simulink model "ROME_9DOF"  (R2026a)
settings: Solver=FixedStepDiscrete  StopTime=T_scaled  FixedStep=dt_9dof  EnableMultiTasking=on
PostLoadFcn:
  | define_constants
model workspace (MAT data in the model file):
  dddwad = 1
values from neighbouring files (symbols this model uses):
  alphas = [5.49778714378 3.92699081699 2.35619449019 0.785398163397]    [9-24-26-15-33_Case_1_data.mat]    (also in define_constants.m = [deg2rad(315), deg2rad(225), deg2rad(135), deg2rad(45)]; scaled_factor_0.1_scenario1.mat; scaled_factor_1.0_scenario1_semimajor0.5.mat; scaled_factor_1.0_scenario1_semimajor10.mat)
  arm_home = [-0.0523598775598 2.21656815003 -0.174532925199 0 -0.471238898038 0]    [9-24-26-15-33_Case_1_data.mat]    (also in define_constants.m = deg2rad([-3.0; -53.0; -10.0; 0.0; -27.0; 0.0]); scaled_factor_0.1_scenario1.mat = [0 -0.5 0.9 0 0.7 0]; scaled_factor_1.0_scenario1_semimajor0.5.mat = [0 -0.5 0.9 0 0.7 0]; scaled_factor_1.0_scenario1_semimajor10.mat = [0 -0.5 0.9 0 0.7 0])
  dist_scale = 0.5    [9-24-26-15-33_Case_1_data.mat]    (also in define_constants.m; scaled_factor_0.1_scenario1.mat = 0.1; scaled_factor_1.0_scenario1_semimajor0.5.mat = 1; scaled_factor_1.0_scenario1_semimajor10.mat = 1)
  dt_9dof = 0.05    [9-24-26-15-33_Case_1_data.mat]    (also in define_constants.m; scaled_factor_0.1_scenario1.mat; scaled_factor_1.0_scenario1_semimajor0.5.mat; scaled_factor_1.0_scenario1_semimajor10.mat)
  elements = [1.4 0.5 0 0 0 0]    [9-24-26-15-33_Case_1_data.mat]    (also in define_constants.m = [1.4, 0.5, 0, 0, 0, 0]; scaled_factor_0.1_scenario1.mat; scaled_factor_1.0_scenario1_semimajor0.5.mat = [0.5 0.5 0 0 0 0]; scaled_factor_1.0_scenario1_semimajor10.mat = [10 0.5 0 0 0 0])
  EnableHardware = 1    [9-24-26-15-33_Case_1_data.mat]    (also in define_constants.m = 0; scaled_factor_0.1_scenario1.mat; scaled_factor_1.0_scenario1_semimajor0.5.mat = 0; scaled_factor_1.0_scenario1_semimajor10.mat = 0)
  EnableMotive = 0    [9-24-26-15-33_Case_1_data.mat]    (also in define_constants.m; scaled_factor_0.1_scenario1.mat; scaled_factor_1.0_scenario1_semimajor0.5.mat; scaled_factor_1.0_scenario1_semimajor10.mat)
  l = 0.35    [9-24-26-15-33_Case_1_data.mat]    (also in define_constants.m; scaled_factor_0.1_scenario1.mat; scaled_factor_1.0_scenario1_semimajor0.5.mat; scaled_factor_1.0_scenario1_semimajor10.mat)
  max_rpm = 60    [9-24-26-15-33_Case_1_data.mat]    (also in define_constants.m = 120)
  mu = 1    [9-24-26-15-33_Case_1_data.mat]    (also in define_constants.m; scaled_factor_0.1_scenario1.mat; scaled_factor_1.0_scenario1_semimajor0.5.mat; scaled_factor_1.0_scenario1_semimajor10.mat)
  par = [0 0 0 0]    [9-24-26-15-33_Case_1_data.mat]    (also in define_constants.m; scaled_factor_0.1_scenario1.mat; scaled_factor_1.0_scenario1_semimajor0.5.mat; scaled_factor_1.0_scenario1_semimajor10.mat)
  q0_9dof = [0.677771808272 -0.00755462438616 -3.12693488796 -0.0377021119487 2.24411564415 -0.258737272647 -2.32231542275e-11 -0.414582044708 -0.0230443461837]    [9-24-26-15-33_Case_1_data.mat]    (also in define_constants.m = ik9_warm_start(q0_9dof, p_ref0, u_ref0); scaled_factor_0.1_scenario1.mat = [0.419801308893 0.000544930315419 0.0507789134473 -0.0492210; scaled_factor_1.0_scenario1_semimajor0.5.mat = [0.597187365937 -0.000238669500436 0.0496562814685 -0.050343; scaled_factor_1.0_scenario1_semimajor10.mat = [5.22393486573 -0.00540150303984 0.0379419048008 -0.06205809)
  qd0_9dof = [0 0 0 0 0 0 0 0 0]    [9-24-26-15-33_Case_1_data.mat]    (also in define_constants.m = zeros(9,1); scaled_factor_0.1_scenario1.mat = [-0.00873270617541 7.41536811609 7.95269754129 7.95269754129; scaled_factor_1.0_scenario1_semimajor0.5.mat = [0.00054251154028 1.74656993429 1.10426548167 1.10426548167 ; scaled_factor_1.0_scenario1_semimajor10.mat = [-0.00013965780749 0.213299087201 -0.0129277229128 -0.012927)
  r = 0.0762    [9-24-26-15-33_Case_1_data.mat]    (also in define_constants.m; scaled_factor_0.1_scenario1.mat; scaled_factor_1.0_scenario1_semimajor0.5.mat; scaled_factor_1.0_scenario1_semimajor10.mat)
  scenario = 1    [9-24-26-15-33_Case_1_data.mat]    (also in define_constants.m; scaled_factor_0.1_scenario1.mat; scaled_factor_1.0_scenario1_semimajor0.5.mat; scaled_factor_1.0_scenario1_semimajor10.mat)
  time_scale = 0.4    [9-24-26-15-33_Case_1_data.mat]    (also in define_constants.m = 0.2; scaled_factor_0.1_scenario1.mat; scaled_factor_1.0_scenario1_semimajor0.5.mat; scaled_factor_1.0_scenario1_semimajor10.mat)
  z_work = 0.32    [9-24-26-15-33_Case_1_data.mat]    (also in define_constants.m = 0.42; scaled_factor_0.1_scenario1.mat = 0.42; scaled_factor_1.0_scenario1_semimajor0.5.mat = 0.42; scaled_factor_1.0_scenario1_semimajor10.mat = 0.42)
libraries: simulink x1
(part 1 of 3)
settings Model: Creator=ke350927  LastModifiedBy=ke350927
settings SolverCC: PositivePriorityOrder=on
settings DebuggingCC: UnderspecifiedInitializationDetection=Classic
settings HardwareCC: ProdBitPerLong=64.0  ProdHWDeviceType=Intel->x86-64 (Linux 64)
settings RTWCC: SystemTargetFile=sldrt.tlc  TemplateMakefile=sldrt.tmf  RTWCompilerOptimization=on  Description=Simulink Desktop Real-Time
settings CodeAppCC: MaxIdLength=95.0
settings SimulinkDesktopRealTimeCC: RealTimeExecution=kernel  ExtModeTransport=0.0  ExtModeStaticAllocSize=1000000.0  TargetLibSuffix=_sldrt.a  TargetPreCompLibLocation=C:\Program Files\MATLAB\R2026a\toolbox\sldrt\lib\win64  MultiwordLength=2048.0  ParMdlRefBuildCompliant=on
settings SimscapeCC: SimscapeLogDecimation=1  SimscapeNominalValues="[{\"value\":\"1\",\"unit\":\"A\"},{\"value\":\"1\",\"unit\":\"bar\"},{\"value\":\"1\",\"unit\":\"cm^2\"},{\"value\":\"1\",\"unit\":\"cm^3/s\"},{\"value\":\"1\",\"unit\":\"kJ/kg\"},{\"value\":\"1\",\"unit\":\"kW\"},{\"value\":\"1\",\"unit\":\"l\"},{\"value\":\"1\",\"unit\":\"N\"},{\"value\":\"1\",\"unit\":\"N*m\"},{\"value\":\"1\",\"unit\":\"V\"}]"  SimscapeLogDataHistory=5000  SimscapeLogType=none

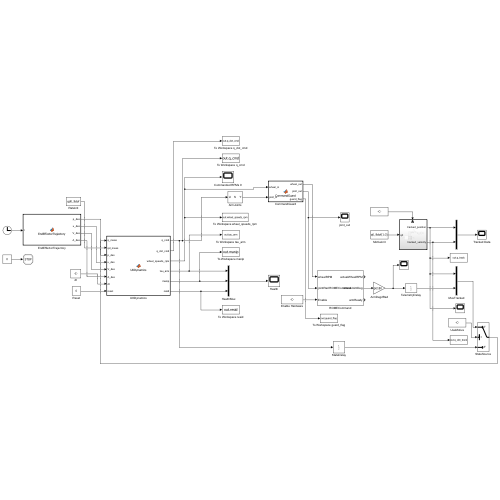
[thumbnail: Simulink's stored preview of the top-level diagram]
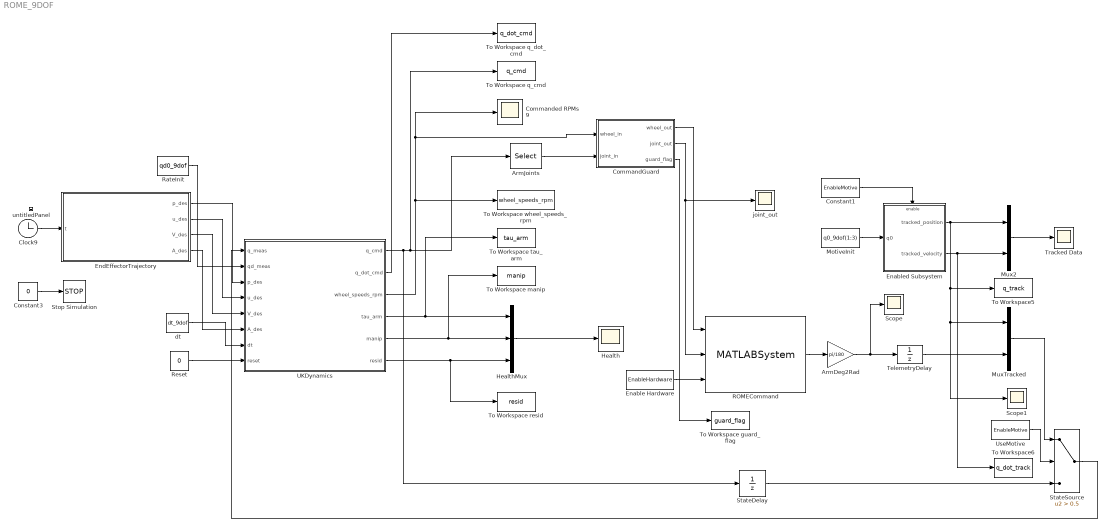
== system ROME_9DOF ==
  ArmDeg2Rad : Gain  Gain=pi/180
  ArmJoints : Selector  InputPortWidth=9  IndexOptions=Index vector (dialog)  Indices=4:9  OutputSizes=1
  Clock9 : Clock
  CommandGuard : MATLAB Function  TreatAsAtomicUnit=on
  Commanded RPMs 9 : Scope
      settings: ActiveDisplayYMinimum=-34.683228987770512  ActiveDisplayYMaximum=56.745429364139078
  Constant1 : Constant  Value=EnableMotive
  Constant3 : Constant  Value=0
  Enable Hardware : Constant  Value=EnableHardware
  Enabled Subsystem : Subsystem  TreatAsAtomicUnit=on
  EndEffectorTrajectory : MATLAB Function  TreatAsAtomicUnit=on
  Health : Scope
      settings: ActiveDisplayYMinimum=-2.44304879075833  ActiveDisplayYMaximum=9.5657314364182238
  HealthMux : Mux  Inputs=3
  MotiveInit : Constant  Value=q0_9dof(1:3)
  Mux2 : Mux  Inputs=2
  MuxTracked : Mux  Inputs=2
  ROMECommand : MATLABSystem  System=ROMECommand  ESP32_IP=192.168.4.1  ESP32_Port=3333  SimulateUsing=Interpreted execution
      mask Type: ROMECommand
  RateInit : Constant  Value=qd0_9dof
  Reset : Constant  Value=0
  Scope : Scope
      settings: ActiveDisplayYMinimum=-0.48446747803384349  ActiveDisplayYMaximum=0.83103253402443622  DataLoggingVariableName=ScopeData3
  Scope1 : Scope
      settings: ActiveDisplayYMinimum=-0.94105790464333883  ActiveDisplayYMaximum=0.87300105227276092
  StateDelay : UnitDelay  InitialCondition=q0_9dof  SampleTime=dt_9dof
  StateSource : Switch  Criteria=u2 > Threshold  Threshold=0.5  SaturateOnIntegerOverflow=off  InputSameDT=off
  Stop Simulation : Stop
  TelemetryDelay : UnitDelay  InitialCondition=arm_home  SampleTime=dt_9dof
  To Workspace guard_flag : ToWorkspace  VariableName=guard_flag  SaveFormat=Timeseries  SampleTime=-1
  To Workspace manip : ToWorkspace  VariableName=manip  SaveFormat=Timeseries  SampleTime=-1
  To Workspace q_cmd : ToWorkspace  VariableName=q_cmd  SaveFormat=Timeseries  SampleTime=-1
  To Workspace q_dot_cmd : ToWorkspace  VariableName=q_dot_cmd  SaveFormat=Timeseries  SampleTime=-1
  To Workspace resid : ToWorkspace  VariableName=resid  SaveFormat=Timeseries  SampleTime=-1
  To Workspace tau_arm : ToWorkspace  VariableName=tau_arm  SaveFormat=Timeseries  SampleTime=-1
  To Workspace wheel_speeds_rpm : ToWorkspace  VariableName=wheel_speeds_rpm  SaveFormat=Timeseries  SampleTime=-1
  To Workspace5 : ToWorkspace  VariableName=q_track  SaveFormat=Timeseries  SampleTime=-1
  To Workspace6 : ToWorkspace  VariableName=q_dot_track  SaveFormat=Timeseries  SampleTime=-1
  Tracked Data : Scope
      settings: ActiveDisplayYMinimum=-1.51772  ActiveDisplayYMaximum=1.20458
  UKDynamics : MATLAB Function  TreatAsAtomicUnit=on
  UseMotive : Constant  Value=EnableMotive
  dt : Constant  Value=dt_9dof
  joint_out : Scope
      settings: ActiveDisplayYMinimum=-0.077149087759822071  ActiveDisplayYMaximum=0.85971146467042214  DataLoggingVariableName=ScopeData2
  untitledPanel : Subsystem  Tag=HiddenForWebPanel  IsWebBlockPanel=on
  wires:
  Clock9/1 -> EndEffectorTrajectory/1(t)
  Constant3/1 -> Stop Simulation/1
  Reset/1 -> UKDynamics/8(reset)
  dt/1 -> UKDynamics/7(dt)
  RateInit/1 -> UKDynamics/2(qd_meas)
  CommandGuard/3(guard_flag) -> To Workspace guard_flag/1
  EndEffectorTrajectory/4(A_des) -> UKDynamics/6(A_des)
  EndEffectorTrajectory/3(V_des) -> UKDynamics/5(V_des)
  EndEffectorTrajectory/1(p_des) -> UKDynamics/3(p_des)
  MotiveInit/1 -> Enabled Subsystem/1(q0)
  EndEffectorTrajectory/2(u_des) -> UKDynamics/4(u_des)
  TelemetryDelay/1 -> MuxTracked/2
  UKDynamics/1(q_cmd) -> ArmJoints/1, To Workspace q_cmd/1, StateDelay/1
  UKDynamics/2(q_dot_cmd) -> To Workspace q_dot_cmd/1
  UKDynamics/3(wheel_speeds_rpm) -> CommandGuard/1(wheel_in), Commanded RPMs 9/1, To Workspace wheel_speeds_rpm/1
  UKDynamics/4(tau_arm) -> HealthMux/1, To Workspace tau_arm/1
  UKDynamics/5(manip) -> HealthMux/2, To Workspace manip/1
  UKDynamics/6(resid) -> HealthMux/3, To Workspace resid/1
  ArmJoints/1 -> CommandGuard/2(joint_in)
  HealthMux/1 -> Health/1
  CommandGuard/1(wheel_out) -> ROMECommand/1
  StateSource/1 -> UKDynamics/1(q_meas)
  UseMotive/1 -> StateSource/2
  Enable Hardware/1 -> ROMECommand/3
  ROMECommand/2 -> ArmDeg2Rad/1
  StateDelay/1 -> StateSource/3
  Mux2/1 -> Tracked Data/1
  Constant1/1 -> Enabled Subsystem/Enable
  MuxTracked/1 -> StateSource/1
  ArmDeg2Rad/1 -> Scope/1, TelemetryDelay/1
  Enabled Subsystem/1(tracked_position) -> Scope1/1, MuxTracked/1, To Workspace5/1, Mux2/1
  Enabled Subsystem/2(tracked_velocity) -> To Workspace6/1, Mux2/2
  CommandGuard/2(joint_out) -> ROMECommand/2, joint_out/1

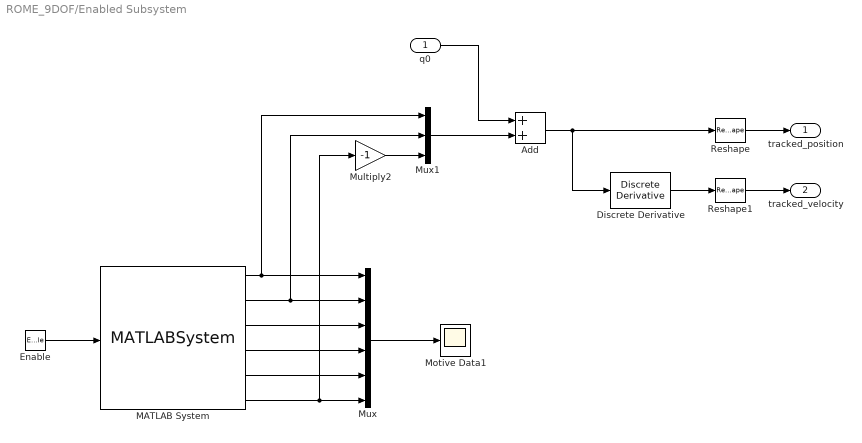
== system ROME_9DOF/Enabled Subsystem ==
  q0 : Inport
  Enable : EnablePort  ShowOutputPort=on
  Add : Sum
  Discrete Derivative : simulink/Discrete/Discrete Derivative  gainval=1.0  ICPrevScaledInput=0.0  OutMin=[]  OutMax=[]  OutDataType=fixdt(1, 16)  OutScaling=2^-10  DoSatur=off
  MATLAB System : MATLABSystem  Priority=1  System=MotiveData  RigidBodyID=1  MulticastIP=239.255.42.99  DataPort=1511  SimulateUsing=Interpreted execution
      mask Type: MotiveData
  Motive Data1 : Scope
      settings: ActiveDisplayYMinimum=-0.0048  ActiveDisplayYMaximum=0.32815  DataLoggingSaveFormat=Array
  Multiply2 : Gain  Gain=-1
  Mux : Mux  Inputs=6
  Mux1 : Mux  Inputs=3
  Reshape : Reshape  OutputDimensionality=Customize  OutputDimensions=[3, 1]
  Reshape1 : Reshape  OutputDimensionality=Customize  OutputDimensions=[3, 1]
  tracked_position : Outport
  tracked_velocity : Outport  Port=2
  wires:
  Discrete Derivative/1 -> Reshape1/1
  MATLAB System/4 -> Mux/4
  MATLAB System/3 -> Mux/3
  MATLAB System/5 -> Mux/5
  MATLAB System/6 -> Mux/6, Multiply2/1
  Mux/1 -> Motive Data1/1
  Enable/1 -> MATLAB System/1
  MATLAB System/2 -> Mux1/2, Mux/2
  MATLAB System/1 -> Mux1/1, Mux/1
  Multiply2/1 -> Mux1/3
  Reshape/1 -> tracked_position/1
  Reshape1/1 -> tracked_velocity/1
  Add/1 -> Discrete Derivative/1, Reshape/1
  Mux1/1 -> Add/2
  q0/1 -> Add/1

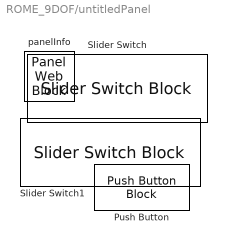
== system ROME_9DOF/untitledPanel ==
  Push Button : PushButtonBlock  Tag=HiddenForWebPanel  PanelInfo="{\"height\":87,\"left\":21,\"panelId\":\"panelId-a39fcf5c-14f9-48cf-a4ef-42f4a30cc727\",\"top\":169,\"type\":\"panelChild\",\"version\":\"2019b\",\"width\":175,\"zIndex\":1500006}"  ButtonText=STOP  Icon=Ex4  IconOnColor=[0.0, 0.39215686274509803, 0.0]  IconOffColor=[0.0, 1.0, 0.0]  OffValue=0.000000
  Slider Switch : SliderSwitchBlock  Tag=HiddenForWebPanel  PanelInfo="{\"height\":68,\"left\":18,\"panelId\":\"panelId-a39fcf5c-14f9-48cf-a4ef-42f4a30cc727\",\"top\":18,\"type\":\"panelChild\",\"version\":\"2019b\",\"width\":180,\"zIndex\":1500004}"
  Slider Switch1 : SliderSwitchBlock  Tag=HiddenForWebPanel  PanelInfo="{\"height\":68,\"left\":17,\"panelId\":\"panelId-a39fcf5c-14f9-48cf-a4ef-42f4a30cc727\",\"top\":93,\"type\":\"panelChild\",\"version\":\"2019b\",\"width\":180,\"zIndex\":1500008}"
  panelInfo : PanelWebBlock  Tag=HiddenForWebPanel  PanelInfo="{\"compacted\":false,\"height\":274,\"isActiveTab\":true,\"left\":1120,\"name\":\"Panel\",\"panelId\":\"panelId-a39fcf5c-14f9-48cf-a4ef-42f4a30cc727\",\"popoutData\":{\"height\":0,\"left\":0,\"maximized\":false,\"top\":0,\"width\":0},\"popoutMode\":\"component\",\"tabIndex\":0,\"tabbedSetId\":\"tabbedSet7305451321\",\"top\":89,\"type\":\"panel\",\"version\":\"2019b\",\"visible\":true,\"width\":214,\"zIndex\":1500002}"  PanelSnapshot=<binary blob, 12168 chars, not shown>
